simulink model "TP_ex3_Simulink"  (R2020b)
settings: Solver=VariableStepAuto  StartTime=0.0  StopTime=10.0  RelTol=1e-3
settings Model: Creator=macbook  LastModifiedBy=macbook

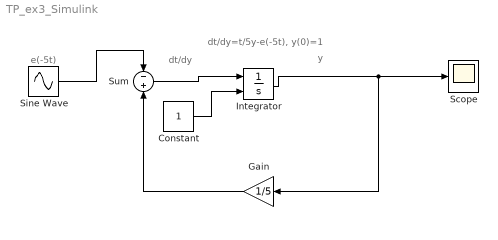
== system TP_ex3_Simulink ==
  note: y
  note: dt/dy
  note: e(-5t)
  note: dt/dy=t/5y-e(-5t), y(0)=1
  Constant : Constant
  Gain : Gain  Gain=1/5
  Integrator : Integrator  InitialConditionSource=external
  Scope : Scope
  Sine Wave : Sin  SampleTime=0
  Sum : Sum  Inputs=-+
  wires:
  Sine Wave/1 -> Sum/1
  Integrator/1 -> Gain/1, Scope/1
  Gain/1 -> Sum/2
  Constant/1 -> Integrator/2
  Sum/1 -> Integrator/1
